simulink model "two_bus_GT"  (R2024b)
settings: Solver=VariableStepAuto  StartTime=0.0  StopTime=20  FixedStep=2e-6  RelTol=1e-3  AbsTol=1e-3  EnableMultiTasking=on
libraries: ee_lib x7, fl_lib x6, nesl_utility x1
CloseFcn:
  | try,close(h1_TwoBusLoadflow),end
  | clear h1_TwoBusLoadflow
  | 
  | clear simlog_TwoBusLoadflow
  | clear logsout_TwoBusLoadflow
Description:
  | 2-Bus Loadflow
settings Model: Creator=The MathWorks, Inc.  LastModifiedBy=xinxing
settings SolverCC: AutoScaleAbsTol=off  AlgebraicLoopSolver=TrustRegion  MaxZcPerStep=1
settings DataIOCC: MaxDataPoints=110000  SaveOutput=off  SignalLogging=off  DSMLogging=off  SaveTime=off  ReturnWorkspaceOutputs=off  SignalLoggingName=logsout_IEEE9BusLoadflow
settings OptimizationCC: ReuseModelBlockBuffer=off  LifeSpan=inf
settings DebuggingCC: UnderspecifiedInitializationDetection=Classic  MergeDetectMultiDrivingBlocksExec=none  MaxConsecutiveZCsMsg=warning  UnconnectedInputMsg=warning  UnconnectedOutputMsg=warning  UnconnectedLineMsg=warning  SFUnexpectedBacktrackingDiag=warning  SFNoUnconditionalDefaultTransitionDiag=warning  SFExecutionAtInitializationDiag=none  ArithmeticOperatorsInVariantConditions=warning
settings ModelReferenceCC: EnableRefExpFcnMdlSchedulingChecks=on
settings SFSimCC: SimUseLocalCustomCode=off
settings RTWCC: RTWUseLocalCustomCode=off  GPUComputeCapability=3.5  DLArmComputeVersion=19.05
settings CodeAppCC: StateflowObjectComments=on
settings GRTTargetCC: TargetLangStandard=C89/C90 (ANSI)
settings ConfigComp: CovMetricSettings=dw  CovSaveCumulativeToWorkspaceVar=on  CovSaveSingleToWorkspaceVar=on  CovExternalEMLEnable=off
settings SimscapeCC: SimscapeNormalizeSystem=off  SimscapeLogType=all  SimscapeLogSimulationStatistics=on  SimscapeLogName=simlog_TwoBusLoadflow

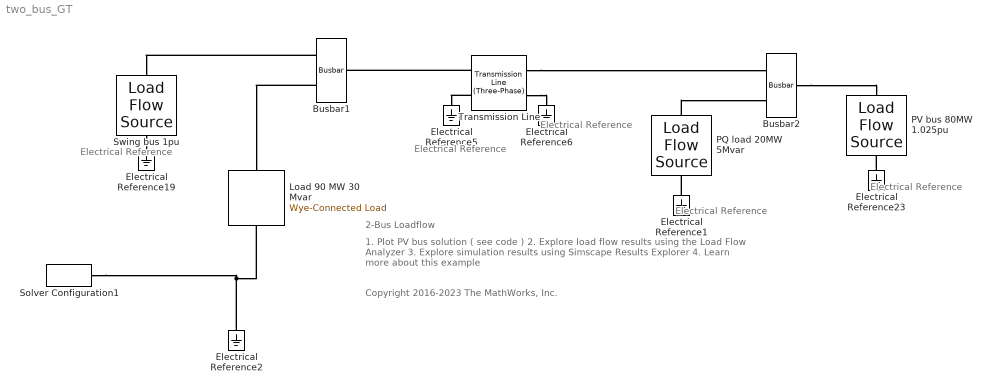
== system two_bus_GT ==
  note: 2-Bus Loadflow
  note: 1. Plot PV bus solution ( see code )
      | 2. Explore load flow results using the Load Flow Analyzer
      | 3. Explore simulation results using Simscape Results Explorer
      | 4. Learn more about this example
  note: Copyright 2016-2023 The MathWorks, Inc.
  note: Electrical
      | Reference
  note: Electrical
      | Reference
  note: Electrical
      | Reference
  note: Electrical
      | Reference
  note: Electrical
      | Reference
  Busbar1 : ee_lib/Connectors & References/Busbar  Tag="1.000 pu\\n0.00 deg\\n30.4   59.6  -90.0 MW\\n7.5   22.5  -30.0 Mvar"  n_nodes=ee.enum.connectors.busbar_number_of_connections.three  VRated=13.8 kV  freq=60 Hz  show_ps=ee.enum.connectors.busbar_measurement.false
      settings: AttributesFormatString=%<Tag>  InternalSimscapePortConfiguration="{\"Bottom\":[],\"Left\":[{\"id\":\"N1\",\"label\":\"~1\",\"type\":\"foundation.electrical.three_phase\"},{\"id\":\"N3\",\"label\":\"~3\",\"type\":\"foundation.electrical.three_phase\"}],\"Right\":[{\"id\":\"N2\",\"label\":\"~2\",\"type\":\"foundation.electrical.three_phase\"}],\"Top\":[]}"
  Busbar2 : ee_lib/Connectors & References/Busbar  Tag="1.025 pu\\n2.51 deg\\n-60.0   80.0  -20.0 MW\\n-25.6   30.6   -5.0 Mvar"  n_nodes=ee.enum.connectors.busbar_number_of_connections.three  VRated=13.8 kV  freq=60 Hz  show_ps=ee.enum.connectors.busbar_measurement.false
      settings: AttributesFormatString=%<Tag>  InternalSimscapePortConfiguration="{\"Bottom\":[],\"Left\":[{\"id\":\"N1\",\"label\":\"~1\",\"type\":\"foundation.electrical.three_phase\"},{\"id\":\"N3\",\"label\":\"~3\",\"type\":\"foundation.electrical.three_phase\"}],\"Right\":[{\"id\":\"N2\",\"label\":\"~2\",\"type\":\"foundation.electrical.three_phase\"}],\"Top\":[]}"
  Electrical Reference{1..2,5..6,19,23} (6 alike) : fl_lib/Electrical/Electrical Elements/Electrical Reference
  Load 90 MW 30 Mvar : ee_lib/Passive/RLC Assemblies/Wye-Connected Load  port_option=ee.enum.threePhasePort.composite  parameterization=2  component_structure=1  component_structure_PQ=4  R=1 Ohm  L=0.001 H  C=1e-6 F  VRated=13.8 kV  FRated=60 Hz  P=90 MW  Qpos=30 MW  Qneg=-100 V*A  R_parasitic=1e-6 Ohm  G_parasitic=1e-6 1/Ohm  R_parasitic_PQ=1e-6 Ohm  G_parasitic_PQ=1e-6*0 1/Ohm  Vmag0=230e3 V  Vang0=0 rad  Freq0=60 Hz  IL_specify=on  IL_priority=High  IL=[ 0 0 0 ] A  IL_nominal_specify=off  IL_nominal_value=1  IL_nominal_unit=A  VC_specify=on  VC_priority=High  VC=[ 0 0 0 ] V  VC_nominal_specify=off  VC_nominal_value=1  VC_nominal_unit=V
  PQ load 20MW 5Mvar : ee_lib/Sources/Load Flow Source  source_type=ee.enum.sources.load_flow_source_type.PQ  v_pu_src=1  active_power_generated=85 MW  active_power_consumed=20 MW  reactive_power_consumed=5 MW  v_pu=1.025  VRated=13.8 kV  freq=60 Hz  shift_src=0 deg  impedance_option=ee.enum.sources.load_flow_source_impedance.None  SShortCircuit=8000 MW  XR=15  R=0.01 Ohm  L=3.97e-4 H  G_parasitic=0 1/Ohm  minimum_pu=0.95  phase_search_range=[-30, 30] deg  I_specify=off  I_priority=None  I=[ 0 0 0 ] A  I_nominal_specify=off  I_nominal_value=1  I_nominal_unit=A  V_impedance_specify=off  V_impedance_priority=None  V_impedance=[ 0 0 0 ] V  V_impedance_nominal_specify=off  V_impedance_nominal_value=1  V_impedance_nominal_unit=V
      settings: InternalSimscapePortConfiguration="{\"Bottom\":[],\"Left\":[{\"id\":\"N\",\"label\":\"~\",\"type\":\"foundation.electrical.three_phase\"}],\"Right\":[{\"id\":\"n\",\"label\":\"n\",\"type\":\"foundation.electrical.electrical\"}],\"Top\":[]}"
  PV bus 80MW 1.025pu : ee_lib/Sources/Load Flow Source  source_type=ee.enum.sources.load_flow_source_type.PV  v_pu_src=1  active_power_generated=80 MW  active_power_consumed=0 W  reactive_power_consumed=0 W  v_pu=1.025  VRated=13.8 kV  freq=60 Hz  shift_src=0 deg  impedance_option=ee.enum.sources.load_flow_source_impedance.XRratio  SShortCircuit=8000 MW  XR=15  R=0.01 Ohm  L=3.97e-4 H  G_parasitic=0 1/Ohm  minimum_pu=0.95  phase_search_range=[-30, 30] deg  I_specify=off  I_priority=None  I=[ 0 0 0 ] A  I_nominal_specify=off  I_nominal_value=1  I_nominal_unit=A  V_impedance_specify=off  V_impedance_priority=None  V_impedance=[ 0 0 0 ] V  V_impedance_nominal_specify=off  V_impedance_nominal_value=1  V_impedance_nominal_unit=V
      settings: InternalSimscapePortConfiguration="{\"Bottom\":[],\"Left\":[{\"id\":\"N\",\"label\":\"~\",\"type\":\"foundation.electrical.three_phase\"}],\"Right\":[{\"id\":\"n\",\"label\":\"n\",\"type\":\"foundation.electrical.electrical\"}],\"Top\":[]}"
  Solver Configuration1 : nesl_utility/Solver Configuration  PhysicalDomain=network_engine_domain  SubClassName=solver  LeftPortType=input  RightPortType=generic  Tones=[]  Harmonics=[]  SimulateNoise=off  Profile=off  UseLocalSampling=off  EnableSwitchedLinearOptims=on  FrequencyDomain=off  UseCCode=off  RelTol=0.001  AbsTol=1e-06  MinStep=1e-09  ToWorkspace=off  RevertToSquareIcSolve=off  NumHomotopyIterations=100  PhasorMode=off  PhasorModeNumHarmonics=1  ConsistencySolver=NEWTON_FTOL  IndexReductionMethod=DerivativeReplacement  DoDC=off  ResidualTolerance=1e-09  ConsistencyTolSource=GLOBAL  ConsistencyAbsTol=0.001  ConsistencyRelTol=0.001  ConsistencyTolFactor=0.001  UseLocalSolver=off  LocalSolverChoice=NE_BACKWARD_EULER_ADVANCER  ResolveIndetEquations=on  FunctionEvalNumThread=1  LocalSolverSampleTime=0.001  DoFixedCost=off  MaxNonlinIter=3  MaxModeIter=2  ComputeImpulses=off  ImpulseIterations=2  LinearAlgebra=auto  LinearAlgebraNumThread=0  EquationFormulation=NE_FREQUENCY_TIME_EF  DelaysMemoryBudget=1024  AutomaticFiltering=on  FilteringTimeConstant=0.001  PartitionStorageMethod=AS_NEEDED  PartitionMemoryBudget=1024  PartitionMethod=ROBUST  MultibodyUseLocalSolver=off  MultibodyLocalSolverChoice=ODE1  MultibodyLocalSolverSampleTime=0.001
  Swing bus 1pu : ee_lib/Sources/Load Flow Source  source_type=ee.enum.sources.load_flow_source_type.Swing  v_pu_src=1  active_power_generated=163 MW  active_power_consumed=0 W  reactive_power_consumed=0 W  v_pu=1  VRated=13.8 kV  freq=60 Hz  shift_src=0 deg  impedance_option=ee.enum.sources.load_flow_source_impedance.None  SShortCircuit=8000 MW  XR=15  R=0.01 Ohm  L=3.97e-4 H  G_parasitic=0 1/Ohm  minimum_pu=0.95  phase_search_range=[-30, 30] deg  I_specify=off  I_priority=None  I=[ 0 0 0 ] A  I_nominal_specify=off  I_nominal_value=1  I_nominal_unit=A  V_impedance_specify=off  V_impedance_priority=None  V_impedance=[ 0 0 0 ] V  V_impedance_nominal_specify=off  V_impedance_nominal_value=1  V_impedance_nominal_unit=V
      settings: InternalSimscapePortConfiguration="{\"Bottom\":[],\"Left\":[{\"id\":\"N\",\"label\":\"~\",\"type\":\"foundation.electrical.three_phase\"}],\"Right\":[{\"id\":\"n\",\"label\":\"n\",\"type\":\"foundation.electrical.electrical\"}],\"Top\":[]}"
  Transmission Line : ee_lib/Passive/Lines/Transmission Line (Three-Phase)  length=1 km  freq=60 Hz  R=0.02 Ohm/km  L=0.5 mH/km  M=0.1 mH/km  Cl=0.3 uF/km  Cg=0.1 uF/km  Rm=0 Ohm/km  ModelTwoSections=ee.enum.enable.no  N=1  InterfacePosition=1 km  N1sec=1  N2sec=1  Access_ground=ee.enum.enable.no  R_parasitic=1e-6 Ohm  G_parasitic=1e-6 1/Ohm
      settings: InternalSimscapePortConfiguration="{\"Bottom\":[],\"Left\":[{\"id\":\"N1\",\"label\":\"~1\",\"type\":\"foundation.electrical.three_phase\"},{\"id\":\"g1\",\"label\":\"g1\",\"type\":\"foundation.electrical.electrical\"}],\"Right\":[{\"id\":\"N2\",\"label\":\"~2\",\"type\":\"foundation.electrical.three_phase\"},{\"id\":\"g2\",\"label\":\"g2\",\"type\":\"foundation.electrical.electrical\"}],\"Top\":[]}"
  connections:
  Swing bus 1pu/RConn1 -- Electrical Reference19/LConn1
  Transmission Line/LConn2 -- Electrical Reference5/LConn1
  Transmission Line/RConn2 -- Electrical Reference6/LConn1
  Electrical Reference23/LConn1 -- PV bus 80MW 1.025pu/RConn1
  Transmission Line/LConn1 -- Busbar1/RConn1
  Busbar2/RConn1 -- PV bus 80MW 1.025pu/LConn1
  Transmission Line/RConn1 -- Busbar2/LConn1
  Busbar1/LConn1 -- Swing bus 1pu/LConn1
  Busbar1/LConn2 -- Load 90 MW 30 Mvar/LConn1
  PQ load 20MW 5Mvar/LConn1 -- Busbar2/LConn2
  Electrical Reference1/LConn1 -- PQ load 20MW 5Mvar/RConn1
  Electrical Reference2/LConn1 -- Solver Configuration1/RConn1 -- Load 90 MW 30 Mvar/RConn1
